simulink model "example_TRYradiationFilter"  (R2018b)
settings: Solver=VariableStepDiscrete  StartTime=90*24*3600  StopTime=95*24*3600  MaxStep=60  RelTol=1e-3  EnableMultiTasking=on
undefined symbols (not defined in the file): path_carnot
libraries: carnot x2
settings Model: Creator=drhf  LastModifiedBy=drhf
settings DataIOCC: LimitDataPoints=on  SaveFormat=Array
settings OptimizationCC: ExpressionDepthLimit=2147483647  LifeSpan=inf
settings DebuggingCC: UnderspecifiedInitializationDetection=Classic  MergeDetectMultiDrivingBlocksExec=none  SolverPrmCheckMsg=warning  StateNameClashWarn=warning  SFUnexpectedBacktrackingDiag=warning  SFNoUnconditionalDefaultTransitionDiag=warning  SFExecutionAtInitializationDiag=none
settings HardwareCC: ProdBitPerPointer=32  ProdBitPerSizeT=32  ProdBitPerPtrDiffT=32  ProdLargestAtomicFloat=None  ProdIntDivRoundTo=Undefined  ProdEndianess=Unspecified  ProdWordSize=32  ProdHWDeviceType=32-bit Generic
settings ModelReferenceCC: PropagateSignalLabelsOutOfModel=off
settings SFSimCC: SimUseLocalCustomCode=off
settings RTWCC: RTWUseLocalCustomCode=off
settings CodeAppCC: StateflowObjectComments=on
settings GRTTargetCC: TargetLangStandard=C89/C90 (ANSI)  GeneratePreprocessorConditionals=Disable all  CombineOutputUpdateFcns=off  GRTInterface=on
settings ConfigComp: CovMetricSettings=dw  CovHtmlReporting=on  CovSaveCumulativeToWorkspaceVar=on  CovSaveSingleToWorkspaceVar=on  CovExternalEMLEnable=off

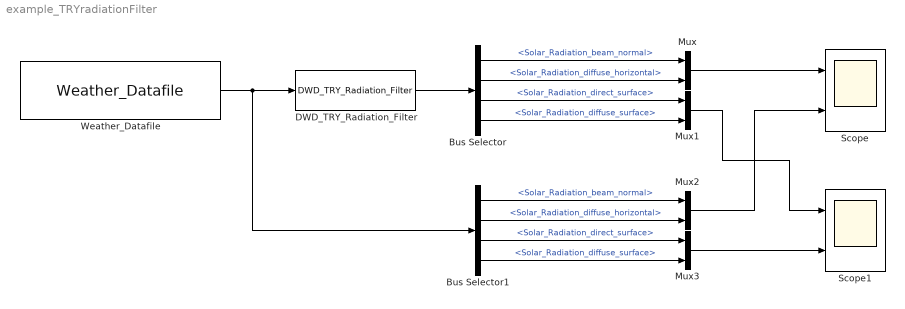
== system example_TRYradiationFilter ==
  Bus Selector : BusSelector  OutputSignals=Solar_Radiation_beam_normal,Solar_Radiation_diffuse_horizontal,Solar_Radiation_direct_surface,Solar_Radiation_diffuse_surface
  Bus Selector1 : BusSelector  OutputSignals=Solar_Radiation_beam_normal,Solar_Radiation_diffuse_horizontal,Solar_Radiation_direct_surface,Solar_Radiation_diffuse_surface
  DWD_TRY_Radiation_Filter : carnot/Weather/DWD_TRY_Radiation_Filter  f=5
  Mux{,1..3} (4 alike) : Mux  Inputs=2
  Scope : Scope  NumInputPorts=2
  Scope1 : Scope  NumInputPorts=2
  Weather_Datafile : carnot/Weather/Weather_Datafile  PathName=path_carnot('data')  FileName='DE_TRY2010_04_averageYear.mat'  UserParam=off  VariableName=DE_TRY2010_04_averageYear  SampleTime=3600
  wires:
  Bus Selector/1 -> Mux/1  "<Solar_Radiation_beam_normal>"
  Bus Selector/2 -> Mux/2  "<Solar_Radiation_diffuse_horizontal>"
  Bus Selector/3 -> Mux1/1  "<Solar_Radiation_direct_surface>"
  Bus Selector/4 -> Mux1/2  "<Solar_Radiation_diffuse_surface>"
  Mux/1 -> Scope/1
  DWD_TRY_Radiation_Filter/1 -> Bus Selector/1
  Bus Selector1/1 -> Mux2/1  "<Solar_Radiation_beam_normal>"
  Bus Selector1/2 -> Mux2/2  "<Solar_Radiation_diffuse_horizontal>"
  Bus Selector1/3 -> Mux3/1  "<Solar_Radiation_direct_surface>"
  Bus Selector1/4 -> Mux3/2  "<Solar_Radiation_diffuse_surface>"
  Weather_Datafile/1 -> DWD_TRY_Radiation_Filter/1, Bus Selector1/1
  Mux2/1 -> Scope/2
  Mux1/1 -> Scope1/1
  Mux3/1 -> Scope1/2
